simulink library "carnot"  (R2013b)
settings: Solver=ode45  StartTime=0.0  StopTime=10.0  RelTol=1e-3
undefined symbols (not defined in the file or in its folder): A, acol, Ahabit, Awin, Azimuth_Angle, AziWin, B, C, c1, c4, capc, caph, CarnotCallbacks_Density, CarnotCallbacks_Enthalpy, CarnotCallbacks_Enthalpy2Temperature, CarnotCallbacks_Entropy, CarnotCallbacks_Evaporation_Enthalpy, CarnotCallbacks_GlobalMessageLevel, CarnotCallbacks_Grashof, CarnotCallbacks_Heat_Capacity, CarnotCallbacks_Kinematic_Viscosity, CarnotCallbacks_Prandtl, CarnotCallbacks_Saturation_Property, CarnotCallbacks_Saturation_Temperature, CarnotCallbacks_Saturation_Value_Water, CarnotCallbacks_Specific_Volume, CarnotCallbacks_Thermal_Conductivity, CarnotCallbacks_Vapour_Content, CarnotCallbacks_Vapour_Pressure, con, cond, d, Dd, density, dfin, dia, DiameterLastPiece, DPConstant, dpipe, DPLinear, DPQuadratic, emission_out, fluid, FluidMix, FluidType, FPC, frame, g, GeodeticHeight, Gwin, heat_capacity, hgt, HP, Hroom, ID, inlet, K, l, lin, lpipe ... (+29)
undefined symbols (not defined in the file): c2, c3, c5, c6, cwall, dactive, height, mc, mID, rho, tau, UAneighbour, UAwall, uloss
libraries: carnot x333, simulink x25, simulink_extras x7
(part 7 of 16)

== system carnot/Source/Heat_Pump ==
  Ground_Source_Heat_Exchanger : Subsystem  mask(vertical ground source heat exchanger){Jahresmitteltemp_C=12, TGrad=0.025, lambdaErde=2.0, cpErde=800, rhoErde=2500, lambdaFill=1.0, cpFill=1000, rhoFill=2000, Sondelaenge=100, B=10, Sondendurchmesser=0.032, Bohrdurchmesser=0.18, sondenfall=1 probe, np=1, DimAxi=10, DimRad=10, Gitterfaktor=2.5}
      mask prompts: Jahresmitteltemp_C "Average annual outdoor temperature  in °C"; TGrad "Temperature gradient in K/m, typical 0.025..0.04"; lambdaErde "Thermal conductivity ground in W/m/K"; cpErde "Heat capacity of the ground in J/kg/K"; rhoErde "Denstiy of the ground in kg/m³"; lambdaFill "Thermal conductivity filling in W/m/K"; cpFill "Heat capacity of the filling in J/kg/K"; rhoFill "Denstiy of the filling in kg/m³"; Sondelaenge "H: Length of earth probe in m"; B "B: probe distance in m"; Sondendurchmesser "Diameter of tube in m"; Bohrdurchmesser "Diameter of drilled hole in m"; sondenfall "Field geometry"; np "Number of parallel tubes"; DimAxi "No. of nodes in axial direction (typical 10)"; DimRad "No. of nodes in radial direction (typical 10)"; Gitterfaktor "grid factor (typical 2.5)"
      mask help:
      | The CARNOT EWS model is a transient model for dynamic simulation of borehole heat exchangers or so-called vertical ground heat exchangers. The model is based on the equations described by [Huber97] and has been implemented using the state space model of Matlab/Simulink [Bianchi06].
      | Bianchi M. A., Adaptive modellbasierte prädiktive Regelung einer Kleinwärmepumenanlage Diss. ETH Zuerich, No. 16892, 2006
      | Huber A, Schuler O., Berechnungsmodul für Erdwärmesonden (EWS). ENET Bericht Nr. 9658807-1, 1997
      mask init:
      | % Sets the parameters for the model
      | % ***********************************************************************
      | % This file is part of the CARNOT Blockset.
      | %   CARNOT is free software: you can redistribute it and/or modify
      | %   it under the terms of the GNU Lesser General Public License as published by
      | %   the Free Software Foundation, either version 3 of the License, or
      | %   (at your option) any later version.
      | %   CARNOT is distributed in the hope that it will be useful,
      | %   but WITHOUT ANY WARRANTY; without even the implied warranty of
      | %   MERCHANTABILITY or FITNESS FOR A PARTICULAR PURPOSE.  See the
      | %   GNU Lesser General Public License for more details.
      | %   You should have received a copy (copying_lesser.txt) of the 
      | %   GNU Lesser General Public License along with CARNOT.  
      | %   If not, see <http://www.gnu.org/licenses/>.
      | %  
      | % **********************************************************************
      | % author list:      fab -> Fabian Ochs
      | %                   hf  -> Bernd Hafner
      | %
      | % version: CarnotVersion.MajorVersionOfFunction.SubversionOfFunction
      | %
      | % Version  Author  Changes                                     Date
      | % 5.1.0    fab     created, based on Diss. Bianchi ETH Zurich  01dec2012
      | % 5.1.1    hf      adapted to carnot input and output struct.  04mar2013 
      | %
      | % Copyright (c) 2012 TU Insbruck, Fabian Ochs
      | 
      | startfall = 2; % 2: g-function
      | mdot = 0.5;
      | teta_in = 1;
      | Massenstrom = mdot/np;
      | Qdot0 = 5000;
      | t_start = 50*8560*3600;
      | 
      | % Geometry
      | Dicke_Sondenrohr = 0.003;
      | lambda_Sondenrohr = 0.48;
      | Bu = .1293;
      | 
      | % Ground Properties
      | aErde = lambdaErde/(rhoErde*cpErde);
      | 
      | % Fluid
      | teta_m = 2; 
      | p0 = 1E5;
      | fluid = 5;
      | mix = 0.25;
      | 
      | Jahresmitteltemp=Jahresmitteltemp_C + 273.15;
      | Bodenerwaermung=1;                          % 0°C
      | Bodentemp=Jahresmitteltemp+Bodenerwaermung; % K
      | 
      | % Calculation
      | lambdaSole=thermal_conductivity(teta_m,p0,fluid,mix);%W/(m K)
      | cpSole=heat_capacity(teta_m,p0,fluid,mix);                                % J/Kg*K
      | rhoSole=density(teta_m,p0,fluid,mix);%kg/m^3
      | vSole=kinematic_viscosity(teta_m,p0,fluid,mix);                             % m2/s
      | 
      | Pr=vSole*rhoSole*cpSole/lambdaSole;
      | rb = Bohrdurchmesser/2;
      | rm = B/2;
      | Rechenradius = rm;
      | Dl=Sondelaenge/DimAxi*2;    
      | 
      | rs=Sondendurchmesser/2;
      | r0 = rs-Dicke_Sondenrohr; % Innenradius
      | r1=Bohrdurchmesser/2;
      | r2=r1+(Rechenradius-r1)*(1-Gitterfaktor)/(1-Gitterfaktor^(DimRad-1))*Gitterfaktor^0;
      | 
      | rz1=((r1^2+r0^2)/2)^0.5;
      | rz2=((r2^2+r1^2)/2)^0.5;
      | 
      | mcpSole=2*cpSole*rhoSole*pi*Dl*(Sondendurchmesser/2)^2;
      | Di = Sondendurchmesser - 2 * Dicke_Sondenrohr;
      | Geschw_Sole= Massenstrom/rhoSole/(Di/2)^2/pi/2; % 2: double U
      | 
      | Vdot = Massenstrom/rhoSole;
      | A_p = (Di/2)^2/pi/2;
      | 
      | Re=Geschw_Sole*Di/vSole;
      | Druckverlust= 1/(1.82*log10(Re)-1.64)^2;
      | K1=1+27.2*Druckverlust/8;
      | K1_o=1.106886;
      | K2=11.7+1.8*Pr^(-1.3);
      | Druckverlust_o=0.031437;
      | St_o= Druckverlust_o/8/(K1_o+K2*(Druckverlust_o/8)^0.5*(Pr^(2/3)-1));
      | Nu_o=St_o*10000*Pr;
      | St= Druckverlust/8/(K1+K2*(Druckverlust/8)^0.5*(Pr^(2/3)-1));
      | 
      | % acc. Hellström    
      | b = Bu/(2*r1);
      | b_max = 1-rs/r1;
      | b_min = rs/r1;
      | sigma = (lambdaFill-lambdaErde)/(lambdaErde+lambdaFill);
      | A = pi*r0^2;
      | vs = Massenstrom/2/rhoSole/A;
      | zeta = 1/((1.82*log10(Re)-1.64)^2);
      | K1 = 1+27.2*zeta/8;
      | K2 = 11.7+1.8*Pr^(-1/3); 
      | R_s = 1/(2*pi*lambda_Sondenrohr)*log(rs/r0);
      |     
      | Nu_turbulent=St*Re*Pr;        
      | Nu_laminar=4.36;
      | 
      | if Re>=10000,
      |     Nu =(zeta/8)*Re*Pr/(K1+K2*(zeta/8)^.5*(Pr^(2/3)-1));
      | elseif Re<10000 && Re>2300
      |     Nu = Nu_laminar*exp(log(Nu_o/Nu_laminar)*log(Re/2300)/log(10000/2300));
      | elseif Re<=2300,
      |     Nu=Nu_laminar;        
      | end
      |     
      | alpha = Nu*lambdaSole/(2*r0);
      | alpha_eff = (1/alpha+r0/lambda_Sondenrohr*log(rs/r0))^-1;
      | alpha0 = lambdaSole/(Di/2*(1-0.5^0.5));
      | alpha0_eff = (1/alpha0+r0/lambda_Sondenrohr*log(rs/r0))^-1;
      | 
      | R_a = 1/(8*pi*alpha*r0);
      | beta = lambdaFill*(1/(r0*alpha)+1/lambda_Sondenrohr*log(rs/r0));
      | 
      | R1_EWS=0.25*(1/(2*pi*alpha_eff*r0*Dl)+1/(2*pi*lambdaFill*Dl)*log((r1-rz1)/r0));
      | R2_EWS=1/(2*pi*Dl)*(1/lambdaFill*log(r1/rz1)+1/lambdaErde*log(rz2/r1));        
      | R10_EWS=0.25*(1/(2*pi*alpha0_eff*r0*Dl)+1/(2*pi*lambdaFill*Dl)*log((r1-rz1)/r0));
      | R20_EWS=1/(2*pi*Dl)*(1/lambdaFill*log(r1/rz1)+1/lambdaErde*log(rz2/r1));        
      | 
      | Ra = 1/(pi*lambdaFill)*(log((2^.5*b*r1)/r0)-1/2*log((2*b*r1)/r0)-1/2*sigma*log((1-b^4)/(1+b^4)))+(1/(2*pi*r0*alpha))+R_s;
      | Rb = (1/(8*pi*lambdaFill))*(beta+log(r1/r0)+log(r1/Bu)+sigma*log(r1^4/(r1^4-Bu^4/16))-(r0^2/Bu^2*(1-sigma*(Bu^474)/(r1^4-Bu^4/16)^2))/((1+beta)/(1-beta)+r0^2/Bu^2*(1+sigma*Bu^4*r1^4/(r1^4-Bu^4/16)^2)));
      | Ra0 = 1/(pi*lambdaFill)*(log((2^.5*b*r1)/r0)-1/2*log((2*b*r1)/r0)-1/2*sigma*log((1-b^4)/(1+b^4)))+(1/(2*pi*r0*alpha0))+R_s;
      | Rb0 = (1/(8*pi*lambdaFill))*(beta+log(r1/r0)+log(r1/Bu)+sigma*log(r1^4/(r1^4-Bu^4/16))-(r0^2/Bu^2*(1-sigma*(Bu^474)/(r1^4-Bu^4/16)^2))/((1+beta)/(1-beta)+r0^2/Bu^2*(1+sigma*Bu^4*r1^4/(r1^4-Bu^4/16)^2)));
      | 
      | if Ra < 4 * Rb
      |     R1 = Ra/(4*Dl);
      |     R2 = (Rb-Ra/4)/Dl+(2*pi*Dl*lambdaErde)^-1*log(rz2/r1);
      |     R10 = Ra0/(4*Dl);
      |     R20 = (Rb0-Ra0/4)/Dl+(2*pi*Dl*lambdaErde)^-1*log(rz2/r1);        
      | else
      |     R1 = R1_EWS;
      |     R2 = R2_EWS;
      |     R10 = R10_EWS;
      |     R20 = R20_EWS;
      | end
      |     
      | % temperaturverlauf axialer richtung
      | L0=cpSole*Massenstrom;      % konstant
      | L00 = 0.0;
      | L1=1/R1;
      | L2=1/R2;
      | L10=1/R10;
      | L20=1/R20;
      | 
      | % matrizen Ad,Bd,Cd,Dd für Tdown
      | Ad=zeros(DimAxi/2,DimAxi/2);
      | Ad0=zeros(DimAxi/2,DimAxi/2);
      | for h=1:DimAxi/2,
      |     Ad(h,h)=-(L0/(mcpSole)+L1/(2*mcpSole));
      |     Ad0(h,h)=-(L00/(mcpSole)+L10/(2*mcpSole));
      | end
      |   
      | for h=1:DimAxi/2-1,
      |     Ad(h+1,h)=L0/(mcpSole);
      |     Ad0(h+1,h)=L00/(mcpSole);
      | end
      | 
      | Bd=zeros(DimAxi/2,DimAxi/2+1);
      | Bd0=zeros(DimAxi/2,DimAxi/2+1);
      | Bd(1,1)=L0/(mcpSole);
      | Bd0(1,1)=L00/(mcpSole);
      | 
      | for h=1:DimAxi/2,
      |     Bd(h,h+1)=L1/(2*mcpSole);
      |     Bd0(h,h+1)=L10/(2*mcpSole);
      | end
      | 
      | Cd=eye(DimAxi/2);
      | Dd=zeros(DimAxi/2,DimAxi/2+1);
      | 
      | % matrizen Au,Bu,Cu,Du für Tup
      | Au=zeros(DimAxi/2,DimAxi/2);
      | Au0=zeros(DimAxi/2,DimAxi/2);
      | for h=1:DimAxi/2,
      |     Au(h,h)=-(L0/(mcpSole)+L1/(2*mcpSole));
      |     Au0(h,h)=-(L00/(mcpSole)+L10/(2*mcpSole));
      | end
      |   
      | for h=1:DimAxi/2-1,
      |     Au(h+1,h)=L0/(mcpSole);
      |     Au0(h+1,h)=L00/(mcpSole);
      | end
      | 
      | Bu=zeros(DimAxi/2,DimAxi/2+1);
      | Bu0=zeros(DimAxi/2,DimAxi/2+1);
      | Bu(1,1)=L0/(mcpSole);
      | Bu0(1,1)=L00/(mcpSole);
      | for h=1:DimAxi/2,
      |     Bu(h,h+1)=L1/(2*mcpSole);
      |     Bu0(h,h+1)=L10/(2*mcpSole);
      | end
      | 
      | Cu=Cd;
      | Du=zeros(DimAxi/2,DimAxi/2+1);
      | 
      | % berechnung von Tradial, von Luzi Valär
      | Dim1=(DimRad-2)*DimAxi/2;
      | r = zeros(1:DimRad);
      | r(1)=Bohrdurchmesser/2;
      | r(2)=r2;
      | for h =3:DimRad,
      |     r(h)=r(h-1)+(Rechenradius-r1)*(1-Gitterfaktor)/(1-Gitterfaktor^(DimRad-1))*Gitterfaktor^(h-2);
      | end
      |     
      | rz = zeros(1:DimRad);
      | rz(1)=((r(1)^2+r0^2)/2)^0.5;
      | for h = 2:DimRad,
      |     rz(h)=((r(h)^2+r(h-1)^2)/2)^0.5;
      | end
      | 
      | L = zeros(1:DimRad);
      | L(1)=L1; 
      | L(2)=L2;
      | for h = 3:DimRad-1,
      |     L(h)=1/(1/(2*pi*Dl)*(1/lambdaErde*log(rz(h)/rz(h-1))));
      | end
      | L(DimRad)=1/(1/(2*pi*Dl)*(1/lambdaErde*log(r(DimRad)/rz(DimRad-1))));
      | 
      | 
      | C = zeros(1:DimRad);
      | C(1)=cpFill*rhoFill*pi*(r(1)^2-4*r0^2)*Dl;
      | for h = 2:DimRad,
      |     C(h)=cpErde*rhoErde*pi*(r(h)^2-r(h-1)^2)*Dl;
      | end
      | 
      | 
      | a=zeros(DimRad-2,DimRad-2);
      | for h = 1:DimRad-2,
      |     a(h,h)=(-L(h)-L(h+1))/C(h);
      | end
      | for h = 1:DimRad-3,
      |     a(h,h+1)=L(h+1)/C(h);
      |     a(h+1,h)=L(h+1)/C(h+1);
      | end
      | 
      | b=zeros(DimRad-2,2);
      |     b(1,1)=L(1)/C(1);
      |     b(DimRad-2,2)=L(DimRad-1)/C(DimRad-2);
      |     
      | %%%%%%%%%%%%%%%%%%%%%%%%%%%%%%%%%%%%%%%%%%%%%%%%%%% 
      |     
      | Ar=a;
      | Ar(DimRad-1:2*(DimRad-2),DimRad-1:2*(DimRad-2))=a;
      |     
      | for h=2:DimAxi/2-1,
      |     Ar(h*(DimRad-2)+1:(h+1)*(DimRad-2),h*(DimRad-2)+1:(h+1)*(DimRad-2))=a;
      | 
      | end  
      | 
      | Br=b;
      | 
      | for h=1:DimAxi/2-1,
      |     Br(h*(DimRad-2)+1:(h+1)*(DimRad-2),2*h+1:2*h+2)=b;   
      | end
      |     
      | 
      | Cr=eye((DimRad-2)*DimAxi/2);
      | Dr=zeros((DimRad-2)*DimAxi/2,DimAxi);
      | 
      | % andere matrizen
      | Cdl=zeros(DimAxi/2,1);
      | Cdl(DimAxi/2,1)=1;
      | Cdl=Cdl';
      | 
      | c1=zeros(DimAxi/2,Dim1);
      | for h=1:DimAxi/2,
      |     c1(1,1)=1;
      |     c1(h,(h-1)*(DimRad-2)+1)=1;
      | end
      | 
      | c31=zeros(1,DimAxi/2);
      | c3(1,1)=1;
      | for h=1:DimAxi/2-1,
      |     c3(1+2*h,1+h)=1;
      | end
      | 
      | c33=zeros(DimAxi,DimAxi/2);
      | c33(1:DimAxi-1,1:DimAxi/2)=c3;
      | 
      | c41=zeros(1,DimAxi/2);
      | c4=c41;
      | c4(2:DimAxi,1:DimAxi/2)=c3;
      | 
      | 
      | % randbedingungen für Tearth,DimRad
      | % anfangsbedingungen für Tradial
      | mu=linspace(0,Sondelaenge,DimAxi/2);
      | T=(mu*TGrad+Bodentemp);
      | Tearth_anf=T'*ones(1,DimRad-2);
      | T_null=Tearth_anf(:,1);
      | teta_fluid_ini = mean(T_null)-273.15;
      | 
      | % anfangsbedingungen für Tdown,Tup
      | Tdown_0=Tearth_anf(:,1);
      | Tup_0=flipud(Tdown_0);
      | Tearth_anf=Tearth_anf';
      | c5=ones(DimAxi/2,1);           
      | 
      | c6=zeros(DimRad-2,3*(DimRad-2));
      | 
      | for i=2:DimRad-2;
      |     c6(1,DimRad-1)=1;
      |     c6(i,DimRad+i-2)=1;
      | end
      | 
      | %% RB
      | Ts_Trichter=7*24*3600; % 7 (1 week according to Huber)
      | Dr_Trichter=1;
      | t_Trichter = linspace(Ts_Trichter,Ts_Trichter*5000,5000);
      | r_Trichter = linspace(Dr_Trichter,Dr_Trichter*20,20);
      | 
      | % g-function
      | xS = [-4 -2 0 2 3];
      | if sondenfall == 1          % 1 Sonde
      |     yS = [4.82 5.69 6.29 6.57 6.6];
      | elseif sondenfall == 2      % 2 Sonden B/H = 0.1
      |     yS = [4.99 6.37 7.62 8.06 8.08];
      | elseif sondenfall == 3      % 2 Sonden B/H = 0.05
      |     yS = [5.30 6.92 8.20 8.67 8.71];
      | elseif sondenfall == 4      % 3x6 Sonden B/H = 0.1
      |     yS = [5.00 9.15 16.40 19.75 20.05];
      | elseif sondenfall == 5      % 5x10 Sonden B/H = 0.1
      |     yS = [5.00 10.2 22.75 29.5 30.05];
      | end
      | 
      | npol = 4;
      | p = polyfit(xS,yS,npol);
      | ts = Sondelaenge^2/(9*aErde);
      | gfunction = zeros(length(t_Trichter),length(r_Trichter));
      | Es = t_Trichter*9*aErde/Sondelaenge^2;
      | 
      | g = polyval(p,log(Es));
      | 
      | for ii = 1:length(r_Trichter)
      |     gfunction(:,ii) = max(0,g - log(r_Trichter(ii)/Sondelaenge/0.0005)); % correction 21-09-2012
      | end
      | 
      | % Startwerte
      | qdot0 = Qdot0/Sondelaenge; 
      | if startfall == 2
      |     Es_start = t_start*9*aErde/Sondelaenge^2;
      |     TEarth0 = zeros(size(Tearth_anf));
      |     for ii = 1:DimAxi/2
      |         for iii = 1:DimRad-1
      |             g_start = polyval(p,log(Es_start));
      |             TEarth0(iii,ii) = Bodentemp + mu(ii)*TGrad - qdot0/(DimAxi/2)*((g_start-log(rz(iii+1)/Sondelaenge/0.0005))/(2*pi*lambdaErde));
      |         end
      |     end    
      | 
      |     T_null = TEarth0(end,:)';
      |     Tearth_anf = TEarth0(1:end-1,:);
      | end
      mask Help: web(['file:///' fullfile(path_carnot('help'),'Ground_Source_Heat_Exchanger.html')],'-helpbrowser')
      mask TypeOptions sondenfall: 1 probe | 2 probes B/H = 0.1 | 2 probes B/H = 0.05 | 3x6 probes B/H = 0.1 | 5x10 probes B/H = 0.1
      mask Display:
      | plot(0,10,100,90,[70,30],[80,80],[35,35,43,43,47,52,57,57,66,66,60,60,54,46,40,40,35],[84,87,87,20,13,13,21,87,87,84,84,20,10,10,20,84,84])
      | port_label('input',1,'THB')
      | port_label('output',1,'THB')
      | port_label('output',2,'Tn')
  HeatPump : Subsystem  mask(heat pump){Tcin=[-5 15], Thout=[35 45 55 60], Qdotc=[14000 12500 10000 9200;26900 24000 21700 20000], Qdoth=[18000 17200 16500 16000;31500 29500 27800 27000], Pel=[4400 5500 7000 7500;4600 6000 7000 7500], caph=80000, capc=50000, UA=7, linc=10, quac=10, linh=10, quah=10}
      mask prompts: Tcin "inlet source temperature vector (°C)"; Thout "outlet load temperature vector (°C)"; Qdotc "source power matrix (W)"; Qdoth "heating power matrix (W)"; Pel "electric power matrix (W)"; caph "thermal capacity hot loop [J/K]"; capc "thermal capacity cold loop [J/K]"; UA "heat loss coefficient [W/K]"; linc "Cold side linear massflow dependant pressure drop in [Pa*s/kg]"; quac "Cold side quadratic massflow dependant pressure drop hot side in [Pa*s²/kg]"; linh "Hot side linear massflow dependant pressure drop in [Pa*s/kg]"; quah "Hot side quadratic massflow dependant pressure drop hot side in [Pa*s²/kg]"
      mask help:
      | Linearized heat pump model. Uses measured data according to EN 14511 as input.
      | heating power: Qdot_h = K1*Tcold_in + K2*Thot_out + K3
      | electric power: Pel = K4*Tcold_in + K5*Thot_out + K6
      | source power: Qdot_c = -K7*Tcold_in - K8*Thot_out - K9
      | differential equation: cap*dTh/dt = Qdot + mdot*cp*(T_in-T) + UA*(Tamb-T)
      | with: cap = mass * heat_capactiy
      | See hp_param.m for the parameters K1 to K9.
      | Literature: Schwamberger, K.: Fortschrittsberichete VDI, Nr. 263, 1991
      mask init:
      | % Matrix construction for hp_param
      | A = reshape(Qdoth',numel(Qdoth),1);
      | A = [A reshape(Qdotc',numel(Qdotc),1)];
      | A = [A reshape(Pel',numel(Pel),1)];
      | Thout_temp = [];
      | Tcin_temp = [];
      | for i=1:numel(Tcin)
      |     for j=1:numel(Thout)
      |         Tcin_temp = [Tcin_temp ; Tcin(i)];
      |     end
      |     Thout_temp = [Thout_temp ; Thout'];
      | end
      | A = [A Tcin_temp Thout_temp];
      | 
      | K = hp_param(A);
      | caph = max(1,caph);
      | capc = max(1,capc);
      mask Help: web(fullfile(path_carnot('help'),'heatpump.html'),'-helpbrowser')
      mask Display:
      | plot(-20,-10,120,110,[10,20,40,60,80,90,90,80,60,40,20,10,10],[60,80,90,90,80,60,40,20,10,10,20,40,60],[40,20],[90,20],[60,80],[90,20],[50,50],[30,50],[60,40],[40,40],[57,43],[33,46],[44,57],[34,46])
      | port_label('input',1,'THB_c')
      | port_label('input',2,'THB_h')
      | port_label('input',3,'Ta')
      | port_label('input',4,'ctr')
      | port_label('output',1,'THB_c')
      | port_label('output',2,'THB_h')
      | port_label('output',3,'HPdat')
  HeatPump_CONF : Subsystem  mask(Heat Pump CONF){parameterfile=DefaultHeatPump}
      mask prompts: parameterfile "Parameter set"
      mask help:
      | Configurated heat pump model, variables are defined in a mat-file (for example in "DefaultHeatPump.mat"). The linearized heat pump model uses measured data (e.g. EN 14511).
      | This block uses predefined parameter sets.
      mask init:
      | % path definitions
      | intpath = fullfile(path_carnot('intlibsl'), 'Source','Heat_Pump', ...
      |     'HeatPump_CONF','parameter_set');
      | pubpath = fullfile(path_carnot('libsl'), 'Source','Heat_Pump', ...
      |     'HeatPump_CONF','parameter_set');
      | 
      | [namelist, lib] = CarnotCallbacks_getConfNamelist(intpath,pubpath);
      | 
      | if ~lib
      |     myMaskStylesVar{1} = ['popup(', namelist,')'];
      |     set_param(gcb, 'MaskStyles', myMaskStylesVar);
      | end
      | 
      | if exist(fullfile(intpath,[parameterfile '.mat']))
      |     load(fullfile(intpath,parameterfile));
      | else
      |     load(fullfile(pubpath,parameterfile));
      | end
      mask Help: web(fullfile(path_carnot('help'),'heatpump.html'),'-helpbrowser')
      mask TypeOptions parameterfile: DefaultHeatPump
      mask Display:
      | % user defined picture file
      | picfile = fullfile(path_carnot('intlibsl'), ...
      |     'Source','Heat_Pump','HeatPump_CONF','parameter_set', ...
      |     'HeatPump_CONF.jpg');
      | 
      | % show public picture
      | plot([10,20,40,60,80,90,90,80,60,40,20,10,10]/100, ...
      |     [60,80,90,90,80,60,40,20,10,10,20,40,60]/100,[40,20]/100,...
      |     [90,20]/100,[60,80]/100,[90,20]/100,[50,50]/100, ...
      |     [30,50]/100,[60,40]/100,[40,40]/100,...
      |     [57,43]/100,[33,46]/100,[44,57]/100,[34,46]/100)
      | 
      | % show internal picture if defined
      | if ~BlockIsInCarnotLibrary    % if not located in library any more
      |     if exist(picfile)
      |         image(imread(picfile), [0.1, 0, 0.8, 1])
      |         set_param(gcb, 'BackgroundColor', 'White')
      |     end
      | end
      | 
      | port_label('input',1,'THB_c')
      | port_label('input',2,'THB_h')
      | port_label('input',3,'Ta')
      | port_label('input',4,'ctr')
      | port_label('output',1,'THB_c')
      | port_label('output',2,'THB_h')
      | port_label('output',3,'HPdat')

== system carnot/Source/Simple ==
  Constant_THB : Subsystem  InitFcn=load('THB.mat');  mask(constant THB){t=40, mdot=0, p=1e5, mID=No Pressure Drop, fluid=Water, mix=0, dia=0.02, hgt=0}
      mask prompts: t "temperature [degree centigrade]"; mdot "massflow [kg/s]"; p "pressure [Pa]"; mID "Calculation mode"; mix "fluid mixture [0..1]"; dia "diameter [m]"; hgt "Static height in m"
      mask help: Create a constant Thermo-Hydraulic-Bus.
      mask init:
      | mix = min(1, max(0, mix));
      | dia = max(dia, 0.001);
      | ID = (mID-1)*10000+1;
      mask Help: web(['file:///' fullfile(path_carnot('help'),'constant_THB.html')],'-helpbrowser')
      mask TypeOptions mID: No Pressure Drop | Pressure Drop from Massflow | Full Pressure Drop with Static Height
      mask TypeOptions fluid: Water | Air | Cotton Oil | Silicone Oil | Water-Glycol Mix | Tyfocor LS | Water (Constant 20°C) | Air (dry+ constant 20°C)
  THB_fixed_T : Subsystem  InitFcn=load('THB.mat');  mask(set temperature in THB){t=60}
      mask prompts: t "temperature in degree Celsuis"
      mask help: Set a constant temperature in the thermo-hydraulic bus.
      mask Help: web(['file:///' fullfile(path_carnot('help'),'THB_fixed_T.html')],'-helpbrowser')
  THB_fixed_mdot : Subsystem  InitFcn=load('THB.mat');  mask(set masssflow in THB){m=10/60}
      mask prompts: m "massflow in kg/s"
      mask help: Set a constant massflow in the thermo-hydraulic vector.
  THB_set_T : Subsystem  InitFcn=load('THB.mat');  mask(set temperature in THB){}
      mask help: Set a variable temperature in the thermo-hydraulic bus.
      mask Help: web(['file:///' fullfile(path_carnot('help'),'THB_set_T.html')],'-helpbrowser')
  THB_set_mdot : Subsystem  InitFcn=load('THB.mat');  mask(set temperature in THB){}
      mask help: Set the mass flow rate in the thermo-hydraulic bus.
      mask Help: web(['file:///' fullfile(path_carnot('help'),'THB_set_mdot.html')],'-helpbrowser')
  create_THB : Subsystem  InitFcn=load('THB.mat');  mask(create THB){p=1e5, fluid=Water, mix=0, dia=0.02, mID=No Pressure Drop}
      mask prompts: p "pressure [Pa]"; mix "fluid mixture [0..1]"; dia "diameter [m]"; mID "Caclulation mode"
      mask help: Block to create a THB with the variable input T and mdot. The other value can be set as constants in the mask.
      mask init:
      | mix = min(1, max(0, mix));
      | dia = max(dia, 0.001);
      | ID = (mID-1)*10000+1;
      mask Help: web(fullfile(path_carnot('help'),'createTHB.html'),'-helpbrowser')
      mask TypeOptions fluid: Water | Air | Cotton Oil | Silicone Oil | Water-Glycol Mix | Tyfocor LS | Water (Constant 20°C) | Air (dry+ constant 20°C)
      mask TypeOptions mID: No Pressure Drop | Pressure Drop from Massflow | Full Pressure Drop with Static Height

== system carnot/Source/Solar_Thermal ==
  Collector_1xN : Subsystem  mask(collector){acol=2.3, len=2, eta0=0.8, u1=3.5, u2=0.02, u3=0, uwind=0, c_col=1e4, lin=10, qua=10, tini=20, nodes=5}
      mask prompts: acol "collector surface (aperture) in [m²]"; len "length between inlet and outlet [m]"; eta0 "optical efficiency [-]"; u1 "linear heat loss coefficient [W/(m²*K)]"; u2 "quadratic heat loss coefficient [W/(m*K)²]"; u3 "radiative loss coefficient [W/(m²*K)]"; uwind "wind dependent heat loss [W/(m²*K*m/s)]"; c_col "effective heat capacity of collector [J/(m²*K)]"; lin "linear pressure drop Pa/(kg/s)"; qua "quadratic  pressure drop Pa/(kg/s)²"; tini "initial temperature [degree Celsius]"; nodes "number of nodes"
      mask help:
      | Model for tested collectors. Enter test results in this mask.
      | Look under mask to change the incidence angle modifier, the pressure drop and the radiation calculation method.
      mask init:
      | acol = max(acol, 0.01);
      | eta0 = max(eta0,0);
      | c_col = max(c_col, 0.1);
      mask Help: web(fullfile(path_carnot('help'),'Collector_1xN.html'),'-helpbrowser')
      mask Display: plot(-10,0,80,78,[10 16 66 60 10],[16 10 60 66 16],[8,13],[8,13],[63,68],[63,68])
  Collector_EN12975 : Subsystem  mask(solar thermal collector EN 12975){acol=2.5, len=2.3, fta=0.8103, c1=3.757, c2=0.0147, c3=0, c4=0, c5=7062, c6=0, kblangle=[0:5:90], KbL=[1.0000    1.0000    0.9999    0.9996    0.9991    0.9982    0.9965  0.9935    0.9886    0.9807    0.9678    0.9473    0.9148    0.8638   0.7846    0.6644    0.4907    0.2599    0.0000], kbtangle=[0:5:90], KbT=[1.00000 1.00000 1.00000 1.00000 1.00000 1.00000 1.00000 1.00000 1.00000 1.00000 1.00000 0.87500 0.75000 0.62500 0.50000 0.37500 0.25000 0.12500 0], Kd=0.92, lin=0, qua=0, tini=20}
      mask prompts: acol "A : collector surface  [m²]"; len "length between inlet and outlet [m]"; fta "F'(TauAlfa)"; c1 "c1 : heat loss coefficient at (Tm-Ta)=0  [W/(m²*K)]"; c2 "c2: temperature dependence of the heat loss coefficient [W/(m*K)²]"; c3 "c3 : wind speed dependence of the heat loss coefficient [J/(m³K)]"; c4 "c4 : sky temperature dependence of the heat loss coefficient [W/(m²K)]"; c5 "c5 : effective thermal capacity [J/(m²K)]"; c6 "c6 : wind dependence of conversion factor [s/m]"; kblangle "Kb(L): angles for longitudinal IAM [degree]"; KbL "Kb(L) : incident angle modifier in longitudinal plane (beam radiation)"; kbtangle "Kb(T): angles for transversal IAM [degree]"; KbT "Kb(T) : incident angle modifier in transversal plane (beam radiation)"; Kd "Kd : Incidence angle modifier diffuse radiation"; lin "linear pressure drop in Pa/(kg/s)"; qua "quadratic pressure drop in Pa/(kg/s)²"; tini "initial temperature [degree centigrade]"
      mask help:
      | Dynamic 1-node collector model according to EN 12975 standard.
      | Energy balance:
      | mdot cp (Tout-Tin) /A = F'(TauAlfa) Kdir Idir + F'(TauAlfa) Kdfu Idfu
      |        - c1 (Tm-Tamb) - c2 (Tm-Tamb)^2 - c3 v_wind (Tm-Ta) - c6 v_wind Iglb
      |        + c4 (ELongwave - sigmaSB*(Tamb+273.15)^4) - c5 dTm/dt
      |
      | Often in test reports the optical efficiency or conversion factor eta0 is given.
      | The correlation for F'(TauAlfa) is:
      | eta0 = F'(TauAlfa) * (Kdir(15°)*0.85 + Kdfu*0.15)
      | or
      | F'(TauAlfa) = eta0 / (Kdir(15°)*0.85 + Kdfu*0.15)
      mask init:
      | acol = max(acol, 0.01);
      | c5 = max(c5, 0.001);
      mask Help: web(fullfile(path_carnot('help'),'collector_en12975.html'),'-helpbrowser')
      mask Display: disp('solar thermal\ncollector\nEN 12975\nIAM-Table')
  Collector_EN12975_CONF : Subsystem  mask(configurated Solar Thermal Collector){parameterfile=DefaultCollector, tini=20, Ncollector=1}
      mask prompts: parameterfile "Parameter set"; tini "Inital temperature in °C"; Ncollector "Number of collectors in parallel"
      mask help:
      | Dynamic 1-node collector model according to EN 12975 standard.
      | This block uses predefined parameter sets.
      mask init:
      | % path definitions
      | intpath = fullfile(path_carnot('intlibsl'), 'Source','Solar_Thermal', ...
      |     'Collector_EN12975_CONF','parameter_set');
      | pubpath = fullfile(path_carnot('libsl'), 'Source','Solar_Thermal', ...
      |     'Collector_EN12975_CONF','parameter_set');
      | 
      | [namelist, lib] = CarnotCallbacks_getConfNamelist(intpath,pubpath);
      | 
      | % set namelist in mask
      | if ~lib
      |     myMaskStylesVar{1} = ['popup(', namelist,')'];
      |     myMaskStylesVar{2} = 'edit';
      |     myMaskStylesVar{3} = 'edit';
      |     set_param(gcb, 'MaskStyles', myMaskStylesVar);
      | end
      | 
      | if exist(fullfile(intpath,[parameterfile '.mat']))
      |     load(fullfile(intpath,parameterfile));
      | else
      |     load(fullfile(pubpath,parameterfile));
      | end
      mask Help: web(fullfile(path_carnot('help'),'collector_en12975.html'),'-helpbrowser')
      mask TypeOptions parameterfile: DefaultCollector | Vitosol200T_SP2A_3m2 | Vitosol200T_SPE_1_6m2 | Vitosol200T_SPE_3_2m2 | Vitosol200T_SPL_200m2 | Vitosol300T_SP3B_3m2
      mask Display:
      | % user defined picture file
      | picfile = fullfile(path_carnot('intlibsl'), ...
      |     'Source','Solar_Thermal','Collector_EN12975_CONF','parameter_set', ...
      |      'Collector_CONF.jpg');
      | 
      | % show public picture
      | disp('solar thermal\ncollector\nEN 12975\nIAM-Table')
      | 
      | % show internal picture if defined
      | if ~BlockIsInCarnotLibrary    % if not located in library any more
      |     if exist(picfile)
      |         image(imread(picfile), [0, 0, 1, 1])
      |         set_param(gcb, 'BackgroundColor', 'White')
      |     end
      | end
      | 
      | % port labels
      | port_label('input',1,'WDB')
      | port_label('input',2,'pos')
      | port_label('input',3,'THB')
      | port_label('output',1,'Cdat')
      | port_label('output',2,'Tsol')
      | port_label('output',3,'THB')
  Collector_EN12975_FlatPlate : Subsystem  mask(collector){acol=2.5, len=2.3, fta=0.8103, c1=3.757, c2=0.0147, c3=0, c4=0, c5=7062, c6=0, b0=0.12, Kd=0.92, lin=0, qua=0, tini=20}
      mask prompts: acol "A : collector surface  [m²]"; len "length between inlet and outlet [m]"; fta "F'(TauAlfa)"; c1 "c1 : heat loss coefficient at (Tm-Ta)=0  [W/(m²*K)]"; c2 "c2: temperature dependence of the heat loss coefficient [W/(m*K)²]"; c3 "c3 : wind speed dependence of the heat loss coefficient [J/(m³K)]"; c4 "c4 : sky temperature dependence of the heat loss coefficient [W/(m²K)]"; c5 "c5 : effective thermal capacity [J/(m²K)]"; c6 "c6 : wind dependence of conversion factor [s/m]"; b0 "b0 : constant for the calculation of the incident angle modifier (direct radiation)"; Kd "Kd : Incidence angle modifier diffuse radiation"; lin "linear pressure drop in Pa/(kg/s)"; qua "quadratic pressure drop in Pa/(kg/s)²"; tini "initial temperature [degree centigrade]"
      mask help:
      | Dynamic 1-node collector model according to EN 12975 standard.
      | Energy balance:
      | mdot cp (Tout-Tin) /A = F'(TauAlfa) Kdir Idir + F'(TauAlfa) Kdfu Idfu
      |        - c1 (Tm-Tamb) - c2 (Tm-Tamb)^2 - c3 v_wind (Tm-Ta) - c6 v_wind Iglb
      |        + c4 (ELongwave - sigmaSB*(Tamb+273.15)^4) - c5 dTm/dt
      |
      | Often in test reports the optical efficiency or conversion factor eta0 is given.
      | The correlation for F'(TauAlfa) is:
      | eta0 = F'(TauAlfa) * (Kdir(15°)*0.85 + Kdfu*0.15)
      | or
      | F'(TauAlfa) = eta0 / (Kdir(15°)*0.85 + Kdfu*0.15)
      mask init:
      | acol = max(acol, 0.01);
      | c5 = max(c5, 0.001);
      mask Help: web(fullfile(path_carnot('help'),'collector_en12975.html'),'-helpbrowser')
      mask Display: disp('solar thermal\ncollector\nEN 12975\nB0-Optics')
  Collector_EN12975_FlatPlate_CONF : Subsystem  mask(configurated Flat Plate Solar Thermal Collector){parameterfile=DefaultCollectorFlatPlate, tini=20, Ncollector=1}
      mask prompts: parameterfile "Parameter set"; tini "Inital temperature in °C"; Ncollector "Number of collectors in parallel"
      mask help:
      | Dynamic 1-node collector model according to EN 12975 standard using the b0 model for flat plate collector optics.
      | This block uses predefined parameter sets.
      mask init:
      | % path definitions
      | intpath = fullfile(path_carnot('intlibsl'), 'Source','Solar_Thermal', ...
      |     'Collector_EN12975_FlatPlate_CONF','parameter_set');
      | pubpath = fullfile(path_carnot('libsl'), 'Source','Solar_Thermal', ...
      |     'Collector_EN12975_FlatPlate_CONF','parameter_set');
      | 
      | [namelist, lib] = CarnotCallbacks_getConfNamelist(intpath,pubpath);
      | 
      | % set namelist in mask
      | if ~lib
      |     myMaskStylesVar{1} = ['popup(', namelist,')'];
      |     myMaskStylesVar{2} = 'edit';
      |     myMaskStylesVar{3} = 'edit';
      |     set_param(gcb, 'MaskStyles', myMaskStylesVar);
      | end
      | 
      | if exist(fullfile(intpath,[parameterfile '.mat']))
      |     load(fullfile(intpath,parameterfile));
      | else
      |     load(fullfile(pubpath,parameterfile));
      | end
      mask Help: web(fullfile(path_carnot('help'),'collector_en12975.html'),'-helpbrowser')
      mask TypeOptions parameterfile: DefaultCollectorFlatPlate
      mask Display:
      | % user defined picture file
      | picfile = fullfile(path_carnot('intlibsl'), ...
      |     'Source','Solar_Thermal','Collector_EN12975_FlatPlate_CONF','parameter_set', ...
      |     'Collector_CONF.jpg');
      | 
      | % show public picture
      | disp('solar thermal\ncollector\nEN 12975\nIAM-Table')
      | 
      | % show internal picture if defined
      | if ~BlockIsInCarnotLibrary    % if not located in library any more
      |     if exist(picfile)
      |         image(imread(picfile), [0, 0, 1, 1])
      |         set_param(gcb, 'BackgroundColor', 'White')
      |     end
      | end
      | 
      | % port labels
      | port_label('input',1,'WDB')
      | port_label('input',2,'pos')
      | port_label('input',3,'THB')
      | port_label('output',1,'Cdat')
      | port_label('output',2,'Tsol')
      | port_label('output',3,'THB')
  Collector_Unglazed : Subsystem  mask(Unglazed flat plate collector){acol=2.33, len=5, fta=0.9, e_sky=0.9, uc0=10, uc1=3, uc0loss=4, uc1loss=1.5, uc0gain=6, uc1gain=1.5, uc1eta0=0.01, hi=100, c_abs=1e4, c_fl=1e2, lin=0, qua=0, tini=20, nodes=2}
      mask prompts: acol "collector surface (aperture) in [m²]"; len "length between inlet and outlet [m]"; fta "absorption coefficient of the absorber [-]"; e_sky "e thermal emissivity of the absorber (0..1)"; uc0 "U0C heat transfer for condensation [W/(m²*K)]"; uc1 "U1C wind dependent heat transfer for condensation [W/(m²*K*m/s)]"; uc0loss "U0L heat transfer for losses [W/(m²*K)]"; uc1loss "U1L wind dependent heat transfer for losses [W/(m²*K*m/s)]"; uc0gain "U0G heat transfer for gains [W/(m²*K)]"; uc1gain "U1G wind dependent heat transfer for gains [W/(m²*K*m/s)]"; uc1eta0 "U1E wind dependancy of optical efficiency in W/(m²*m/s)"; hi "HI heat transfer between collector and tube [W/(m2.K)]"; c_abs "effective heat capacity of absorber [J/(m²*K)]"; c_fl "effective heat capacity of fluid [J/(m²*K)]"; lin "linear pressure drop in Pa/(kg/s)"; qua "quadratic pressure drop in Pa/(kg/s)²"; tini "initial temperature [degree centigrade]"; nodes "number of nodes (>=2)"
      mask help:
      | 2xN-nodes model:
      | c_abs*dTp/dt=qdot_solar-qdot_conv_gain-qdot_conv_loss-qdot_cond
      |             -qdot_sky-qdot_fluid
      | qdot_solar = absorbed_solar_radiation - U1E*Iglb*vwind
      | qdot_conv_gain = fconv * (U0G + U1G*vwind)*(Tp - Tamb)
      | qdot_conv_loss = (1-fconv)*(U0L + U1L*vwind)*(Tp - Tamb)
      | qdot_cond = fcond*(U0C + U1C*vwind)*ccond*(ps(Tdew) - ps(Tp))
      | qdot_sky = e * const_sigma*(Tp^4 - Tsky^4)
      | qdot_fluid = HI*(Tp-Tfluid)
      | fconv = 1 if Tp > Tamb, 0 otherwise
      | fcond = 1 if Tp below dewpoint, 0 otherwise
      | Look under mask to change the incidence angle modifier, the pressure drop and the radiation calculation method.
      mask init:
      | acol = max(acol, 0.01);
      | fta = max(fta,0);
      | inv_c_abs = 1/max(c_abs,1);
      | inv_c_fl = 1/max(c_fl,1);
      mask Help: web(fullfile(path_carnot('help'),'Collector_Unglazed.html'),'-helpbrowser')
      mask Display: plot(-30,-30,130,120,[0,70,70,0,0],[-0,-0,5,5,-0],[30,30,100,100,30],[100,94,94,100,100],[32,1],[94,5],[40,10],[94,5],[49,19],[94,5],[57,27],[94,5],[65,35],[94,5],[73,43],[94,5],[82,51],[94,5],[90,60],[94,5],[98,68],[94,5])
  Collector_Unglazed_CONF : Subsystem  mask(configurated Solar Thermal Collector){parameterfile=DefaultCollectorUnglazed, tini=20, Ncollector=1}
      mask prompts: parameterfile "Parameter set"; tini "Inital temperature in °C"; Ncollector "Number of collectors in parallel"
      mask help:
      | Dynamic 1-node collector model according to EN 12975 standard.
      | This block uses predefined parameter sets.
      mask init:
      | % path definitions
      | intpath = fullfile(path_carnot('intlibsl'), 'Source','Solar_Thermal', ...
      |     'Collector_Unglazed_CONF','parameter_set');
      | pubpath = fullfile(path_carnot('libsl'), 'Source','Solar_Thermal', ...
      |     'Collector_Unglazed_CONF','parameter_set');
      | 
      | [namelist, lib] = CarnotCallbacks_getConfNamelist(intpath,pubpath);
      | 
      | % set namelist in mask
      | if ~lib
      |     myMaskStylesVar{1} = ['popup(', namelist,')'];
      |     myMaskStylesVar{2} = 'edit';
      |     myMaskStylesVar{3} = 'edit';
      |     set_param(gcb, 'MaskStyles', myMaskStylesVar);
      | end
      | 
      | if exist(fullfile(intpath,[parameterfile '.mat']))
      |     load(fullfile(intpath,parameterfile));
      | else
      |     load(fullfile(pubpath,parameterfile));
      | end
      mask Help: web(fullfile(path_carnot('help'),'Collector_Unglazed.html'),'-helpbrowser')
      mask TypeOptions parameterfile: DefaultCollectorUnglazed
      mask Display:
      | % user defined picture file
      | picfile = fullfile(path_carnot('intlibsl'), ...
      |     'Source','Solar_Thermal','Collector_Unglazed_CONF','parameter_set', ...
      |      'Collector_CONF.jpg');
      | 
      | % show internal picture if defined
      | if ~BlockIsInCarnotLibrary ...      % if not located in library any more
      |         && exist(picfile,'file')    % AND picfile is present
      |     image(imread(picfile), [0.15 0.1 0.7 0.8])
      |     set_param(gcb, 'BackgroundColor', 'White')
      | else
      |     % show public picture
      |     plot([0,70,70,0,0]/100,[-0,-0,5,5,-0]/100,[30,30,100,100,30]/100,...
      |         [100,94,94,100,100]/100,[32,1]/100,[94,5]/100,[40,10]/100,...
      |         [94,5]/100,[49,19]/100,[94,5]/100,[57,27]/100,[94,5]/100,[65,35]/100,...
      |         [94,5]/100,[73,43]/100,[94,5]/100,[82,51]/100,[94,5]/100,[90,60]/100,...
      |         [94,5]/100,[98,68]/100,[94,5]/100)
      |     set_param(gcb, 'BackgroundColor', 'Yellow')
      | end
      | 
      | % port labels
      | port_label('input',1,'WDB')
      | port_label('input',2,'pos')
      | port_label('input',3,'THB')
      | port_label('output',1,'Cdat')
      | port_label('output',2,'Tsol')
      | port_label('output',3,'THB')
  IncidenceAngleModifier : Subsystem
      mask Display: plot(0,0,100,100,[10,10,40,40,10],[10,40,40,10,10],[50,70,90,50],[30,65,30,30],[20,10,10,20,30,40,40,30,20],[50,60,70,80,80,70,60,50,50])
  PressureDropCollector : Subsystem
      mask Display: plot(0,0,100,100,[10,10,40,40,10],[10,40,40,10,10],[50,70,90,50],[30,65,30,30],[20,10,10,20,30,40,40,30,20],[50,60,70,80,80,70,60,50,50])

== system carnot/Source/Ventilation ==
  Constant_AIV : Subsystem  mask(constant AIV){Tsens=20, Tcon=20, Trad=20, mw=0.012, mco=0.01, rhoair=1.2, cpair=1004, pair=100000, nair=0.5}
      mask prompts: Tsens "sensitive temperature [degree centigrade]"; Tcon "convective room temperature [degree centigrade]"; Trad "radiative room temperature [degree centigrade]"; mw "mass of water per mass of air [kgw/kga]"; mco "mass of CO2 per mass of air"; rhoair "density of air in the room [kg/m3]"; cpair "heat capacity of air in the room [J/kgK]"; pair "air pressure in the room [Pa]"; nair "air exchange rate [1/h]"
      mask help: Create a constant Air Infiltration Ventilation Vector (AIV). The AIV is used by the building model (see /Load/Houses/Room_Radiator).
  Ventilation : Subsystem  mask(ventilation system with heat recovery){vent=vent, rec=rec, Vhouse=Ahabit*Hroom}
      mask prompts: vent "ventilation rate in 1/h"; rec "heat recovery (0..1)"; Vhouse "Volume of the house"
      mask help: Mechanical ventilation system with heat recovery for the simple building model (see /Load/Houses/Simpe_House).
      mask init:
      | rec = max(0,min(1,rec));
      mask Help: web(fullfile(path_carnot('help'),'Ventilation.html'),'-helpbrowser')
  Ventilation_AIV : Subsystem  mask(ACTIVE COMPONENT){co2=400}
      mask prompts: co2 "CO2 content of air in ppm"
      mask help:
      | This block represents the AIR VENTILATION from outdoors into a zone.
      |
      | r : rate of nominal air flow between outdoors and indoor, [0,1]
      | [S] : vector for sinks and sources.
      |
      | NOTE: Mass flows of water and CO2 are taken into consideration.
      |
      | ASSUMPTION:
      | Incoming air volume flow is identical to outgoing air volume flow.
      mask init:
      | CO2norm = co2*1e-6;
      mask Help: web(fullfile(path_carnot('help'),'Ventilation_AIV.html'),'-helpbrowser')
      mask Display:
      | plot([0.2 0.35], [0.8 0.7])
      | plot([0.35 0.65], [0.7 0.7])
      | plot([0.65 0.8], [0.7 0.8])
      | plot([0.65 0.8], [0.76 0.8])
      | plot([0.7 0.8], [0.65 0.8])
      | 
      | plot([0.2 0.35], [0.2 0.3])
      | plot([0.35 0.65], [0.3 0.3])
      | plot([0.65 0.8], [0.3 0.2])
      | plot([0.2 0.25], [0.2 0.32])
      | plot([0.2 0.35], [0.2 0.23])
      | 
      | plot ([0.45 0.45], [0 1])
      | plot ([0.55 0.55], [0 1])
      | 
      | plot ([0.45 0.55], [0.2 0.2])
      | plot ([0.45 0.55], [0.8 0.8])
      | 
      | plot ([0.45 0.55], [0 0.2])
      | plot ([0.45 0.55], [0.8 1])
  Ventilation_Window : Subsystem  mask(Ventilation with Heat Recovery and Window){vent=vent, rec=rec, Vhouse=Ahabit*Hroom}
      mask prompts: vent "Ventilation rate in 1/h"; rec "Heat recovery in 0..1"; Vhouse "Volume of the house"
      mask help:
      | Model of a mechanical ventilation system with heat recovery and a ventilation with windows.
      | The is suitable for the simple building model (see /Load/Houses/Simpe_House).
      mask init:
      | rec = max(0, min(1, rec));
      mask Help: web(fullfile(path_carnot('help'),'Ventilation_Window.html'),'-helpbrowser')
      mask Display: plot(0,10,90,80,[20 70 70 20 20],[20 20 70 70 20],[20 70 80 30 20],[20 20 65 65 20])
